simulink model "four_balloons"  (R2020b)
settings: Solver=VariableStepAuto  StartTime=0.0  StopTime=60*5  FixedStep=0.001  RelTol=1e-3
InitFcn:
  | seed1 = randi(100000);
  | seed2 = randi(200000);
model workspace (MAT data in the model file):
  dCoupling = 10
  kCoupling = 10
values from neighbouring files (symbols this model uses):
  Cd = a(4)    [comparisonPlot.m]    (also in optimiseB2.m = 0.185; optimiseBO.m = 0.185; params2.m = 0.185; sim_2balloon.m = 0.185)
  nH = x2nn.nH    [optimiseB2.m]    (also in optimiseBO.m = x.nH; params2.m = 10; sim_2balloon.m = x(2); sim_balloon.m = x(2))
  normalScaling = x2ll.normalScaling    [optimiseB2.m]    (also in optimiseBO.m = x.normalScaling; params2.m = 1; sim_2balloon.m = 0.259830816053; sim_balloon.m = x(5))
  nS = 1    [comparisonPlot.m]    (also in optimiseB2.m = x2nn.nS; optimiseBO.m = x.nS; params2.m = 0.025; sim_2balloon.m = x(3))
  nV = a(7)    [comparisonPlot.m]    (also in optimiseB2.m = x2nn.nV; optimiseBO.m = x.nV; params2.m = 0.5; sim_2balloon.m = x(1))
  rn = a(1)    [comparisonPlot.m]    (also in optimiseB2.m = 0.0625; optimiseBO.m = 0.0625; params2.m = 0.0625; sim_2balloon.m = 0.0625)
  seedX = randi(100000)    [optimiseB2.m]    (also in optimiseBO.m; params2.m; sim_2balloon.m; sim_balloon.m)
  seedX1 = randi(100000)    [optimiseB2.m]    (also in params2.m; sim_2balloon.m)
  seedY = randi(100000)    [optimiseB2.m]    (also in optimiseBO.m; params2.m; sim_2balloon.m; sim_balloon.m)
  seedY1 = randi(100000)    [optimiseB2.m]    (also in params2.m; sim_2balloon.m)
  seedZ = randi(100000)    [optimiseB2.m]    (also in optimiseBO.m; params2.m; sim_2balloon.m; sim_balloon.m)
  seedZ1 = randi(100000)    [optimiseB2.m]    (also in params2.m; sim_2balloon.m)
  theta = a(2)    [comparisonPlot.m]    (also in extract3D.m = deg2rad(-5); optimiseB2.m = x2ll.theta; optimiseBO.m = x.theta; params2.m = 3.5)
  V0 = a(3)    [comparisonPlot.m]    (also in optimiseB2.m = x2ll.V0; optimiseBO.m = x.V0; params2.m = 3.7; sim_2balloon.m = 1.01295922371)
libraries: nesl_utility x37, sm_lib x18, eeGeneralControl x12
(part 2 of 2)

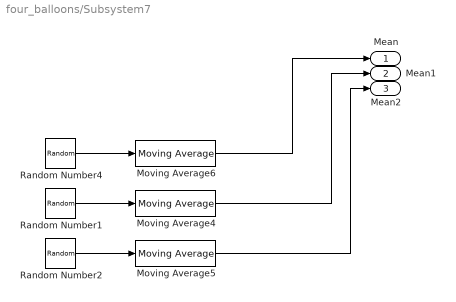
== system four_balloons/Subsystem7 ==
  Moving Average4 : eeGeneralControl/Moving Average  VariantControl=Variant1  LabelModeActiveChoice=Discrete  f=10  x0=0  Ts=nS/10
      settings: SourceProductBaseCode=PS
  Moving Average5 : eeGeneralControl/Moving Average  VariantControl=Variant1  LabelModeActiveChoice=Discrete  f=10  x0=0  Ts=nS/10
      settings: SourceProductBaseCode=PS
  Moving Average6 : eeGeneralControl/Moving Average  VariantControl=Variant1  LabelModeActiveChoice=Discrete  f=10  x0=0  Ts=nS/10
      settings: SourceProductBaseCode=PS
  Random Number1 : RandomNumber  Variance=nH  Seed=seedY1  SampleTime=nS
  Random Number2 : RandomNumber  Variance=nV  Seed=seedZ1  SampleTime=nS
  Random Number4 : RandomNumber  Variance=nH  Seed=seedX1  SampleTime=nS
  " Mean" : Outport
  " Mean1" : Outport  Port=2
  " Mean2" : Outport  Port=3
  wires:
  Moving Average4/1 -> " Mean1"/1
  Moving Average6/1 -> " Mean"/1
  Random Number4/1 -> Moving Average6/1
  Moving Average5/1 -> " Mean2"/1
  Random Number2/1 -> Moving Average5/1
  Random Number1/1 -> Moving Average4/1

== matlab function four_balloons/Subsystem6/Vertical dynamics ==
  data: fx output; sx output; fy output; sy output; x input; xdot input; y input; ydot input; z input; fz output; zdot input; parameters input; sz output

function [fx,sx,fy,sy,fz,sz] = fcn(x,xdot,y,ydot,z,zdot,parameters)

Cd = parameters(1);
rb = parameters(2);
rn = parameters(3);
theta = deg2rad(parameters(4)); 
V0 = parameters(5); 
normalScaling = parameters(6); 

%% Vertical forces

%Horizontal plane displacement
[rotation, rDisplacement] = cart2pol(x,y);

%flow radius
rFlow = rn+z*tan(theta);

%Peak flow velocity
meanFlowVelocity = V0*rn^2/(rFlow)^2;

%Velocity under ball
vFlowActual = flowSpeed(meanFlowVelocity,normalScaling*rFlow,rDisplacement);

%Relative
relativeVelocity = vFlowActual - zdot;

reZ = (1.22 * abs(relativeVelocity) * 2*rb)/(1.81*10^-5);

%Force
fz = sign(rFlow) * 0.5 * Cd * (pi * rb^2) * 1.22 * relativeVelocity^2;

%% Horizontal X forces

innerR = abs(x)-rb;
outerR = abs(x)+rb;
vInner = flowSpeed(meanFlowVelocity,normalScaling*rFlow,innerR);
vOuter = flowSpeed(meanFlowVelocity,normalScaling*rFlow,outerR);
fx = 0.5*1.22*(vOuter^2-vInner^2)*sign(x);

%% Horizontal Y forces
innerR = abs(y)-rb;%3*rb/8;
outerR = abs(y)+rb;%3*rb/8;
vInner = flowSpeed(meanFlowVelocity,normalScaling*rFlow,innerR);
vOuter = flowSpeed(meanFlowVelocity,normalScaling*rFlow,outerR);
fy = 0.5*1.22*(vOuter^2-vInner^2)*sign(y);

%% Drag
dragX = 0.5 * Cd * pi * rb^2 * 1.22 * xdot;
fx = fx - dragX;

dragY = 0.5 * Cd * pi * rb^2 * 1.22 * ydot;
fy = fy - dragY;

%% Force scalings
sx = flowSpeed(meanFlowVelocity,normalScaling*rFlow,x)/flowSpeed(meanFlowVelocity,rFlow,0);
sy = flowSpeed(meanFlowVelocity,normalScaling*rFlow,y)/flowSpeed(meanFlowVelocity,rFlow,0);
sz = flowSpeed(meanFlowVelocity,normalScaling*rFlow,rDisplacement)/flowSpeed(meanFlowVelocity,rFlow,0);

== matlab function four_balloons/Subsystem2/Vertical dynamics ==
  data: fx output; sx output; fy output; sy output; x input; xdot input; y input; ydot input; z input; fz output; zdot input; parameters input; sz output; relativeVelocity output
function [fx,sx,fy,sy,fz,sz, relativeVelocity] = fcn(x,xdot,y,ydot,z,zdot,parameters)

Cd = parameters(1);
rb = parameters(2);
rn = parameters(3);
theta = deg2rad(parameters(4)); 
V0 = parameters(5); 
normalScaling = parameters(6); 

%% Vertical forces

%Horizontal plane displacement
[rotation, rDisplacement] = cart2pol(x,y);

%flow radius
rFlow = rn+z*tan(theta);

%Peak flow velocity
meanFlowVelocity = V0*rn^2/(rFlow)^2;

%Velocity under ball
vFlowActual = flowSpeed(meanFlowVelocity,normalScaling*rFlow,rDisplacement);

%Relative
relativeVelocity = vFlowActual - zdot;

reZ = (1.22 * abs(relativeVelocity) * 2*rb)/(1.81*10^-5);

%Force
fz = sign(rFlow) * 0.5 * Cd * (pi * rb^2) * 1.22 * relativeVelocity^2;

%% Horizontal X forces

innerR = abs(x)-rb;
outerR = abs(x)+rb;
vInner = flowSpeed(meanFlowVelocity,normalScaling*rFlow,innerR);
vOuter = flowSpeed(meanFlowVelocity,normalScaling*rFlow,outerR);
fx = 0.5*1.22*(vOuter^2-vInner^2)*sign(x);

%% Horizontal Y forces
innerR = abs(y)-rb;%3*rb/8;
outerR = abs(y)+rb;%3*rb/8;
vInner = flowSpeed(meanFlowVelocity,normalScaling*rFlow,innerR);
vOuter = flowSpeed(meanFlowVelocity,normalScaling*rFlow,outerR);
fy = 0.5*1.22*(vOuter^2-vInner^2)*sign(y);

%% Drag
dragX = 0.5 * Cd * pi * rb^2 * 1.22 * xdot;
fx = fx - dragX;

dragY = 0.5 * Cd * pi * rb^2 * 1.22 * ydot;
fy = fy - dragY;

%% Force scalings
sx = flowSpeed(meanFlowVelocity,normalScaling*rFlow,x)/flowSpeed(meanFlowVelocity,rFlow,0);
sy = flowSpeed(meanFlowVelocity,normalScaling*rFlow,y)/flowSpeed(meanFlowVelocity,rFlow,0);
sz = flowSpeed(meanFlowVelocity,normalScaling*rFlow,rDisplacement)/flowSpeed(meanFlowVelocity,rFlow,0);

== matlab function four_balloons/Subsystem1/Vertical dynamics ==
  data: fx output; sx output; fy output; sy output; x input; xdot input; y input; ydot input; z input; fz output; zdot input; parameters input; sz output

function [fx,sx,fy,sy,fz,sz] = fcn(x,xdot,y,ydot,z,zdot,parameters)

Cd = parameters(1);
rb = parameters(2);
rn = parameters(3);
theta = deg2rad(parameters(4)); 
V0 = parameters(5); 
normalScaling = parameters(6); 

%% Vertical forces

%Horizontal plane displacement
[rotation, rDisplacement] = cart2pol(x,y);

%flow radius
rFlow = rn+z*tan(theta);

%Peak flow velocity
meanFlowVelocity = V0*rn^2/(rFlow)^2;

%Velocity under ball
vFlowActual = flowSpeed(meanFlowVelocity,normalScaling*rFlow,rDisplacement);

%Relative
relativeVelocity = vFlowActual - zdot;

reZ = (1.22 * abs(relativeVelocity) * 2*rb)/(1.81*10^-5);

%Force
fz = sign(rFlow) * 0.5 * Cd * (pi * rb^2) * 1.22 * relativeVelocity^2;

%% Horizontal X forces

innerR = abs(x)-rb;
outerR = abs(x)+rb;
vInner = flowSpeed(meanFlowVelocity,normalScaling*rFlow,innerR);
vOuter = flowSpeed(meanFlowVelocity,normalScaling*rFlow,outerR);
fx = 0.5*1.22*(vOuter^2-vInner^2)*sign(x);

%% Horizontal Y forces
innerR = abs(y)-rb;%3*rb/8;
outerR = abs(y)+rb;%3*rb/8;
vInner = flowSpeed(meanFlowVelocity,normalScaling*rFlow,innerR);
vOuter = flowSpeed(meanFlowVelocity,normalScaling*rFlow,outerR);
fy = 0.5*1.22*(vOuter^2-vInner^2)*sign(y);

%% Drag
dragX = 0.5 * Cd * pi * rb^2 * 1.22 * xdot;
fx = fx - dragX;

dragY = 0.5 * Cd * pi * rb^2 * 1.22 * ydot;
fy = fy - dragY;

%% Force scalings
sx = flowSpeed(meanFlowVelocity,normalScaling*rFlow,x)/flowSpeed(meanFlowVelocity,rFlow,0);
sy = flowSpeed(meanFlowVelocity,normalScaling*rFlow,y)/flowSpeed(meanFlowVelocity,rFlow,0);
sz = flowSpeed(meanFlowVelocity,normalScaling*rFlow,rDisplacement)/flowSpeed(meanFlowVelocity,rFlow,0);

== matlab function four_balloons/Subsystem4/Vertical dynamics ==
  data: fx output; sx output; fy output; sy output; x input; xdot input; y input; ydot input; z input; fz output; zdot input; parameters input; sz output

function [fx,sx,fy,sy,fz,sz] = fcn(x,xdot,y,ydot,z,zdot,parameters)

Cd = parameters(1);
rb = parameters(2);
rn = parameters(3);
theta = deg2rad(parameters(4)); 
V0 = parameters(5); 
normalScaling = parameters(6); 

%% Vertical forces

%Horizontal plane displacement
[rotation, rDisplacement] = cart2pol(x,y);

%flow radius
rFlow = rn+z*tan(theta);

%Peak flow velocity
meanFlowVelocity = V0*rn^2/(rFlow)^2;

%Velocity under ball
vFlowActual = flowSpeed(meanFlowVelocity,normalScaling*rFlow,rDisplacement);

%Relative
relativeVelocity = vFlowActual - zdot;

reZ = (1.22 * abs(relativeVelocity) * 2*rb)/(1.81*10^-5);

%Force
fz = sign(rFlow) * 0.5 * Cd * (pi * rb^2) * 1.22 * relativeVelocity^2;

%% Horizontal X forces

innerR = abs(x)-rb;
outerR = abs(x)+rb;
vInner = flowSpeed(meanFlowVelocity,normalScaling*rFlow,innerR);
vOuter = flowSpeed(meanFlowVelocity,normalScaling*rFlow,outerR);
fx = 0.5*1.22*(vOuter^2-vInner^2)*sign(x);

%% Horizontal Y forces
innerR = abs(y)-rb;%3*rb/8;
outerR = abs(y)+rb;%3*rb/8;
vInner = flowSpeed(meanFlowVelocity,normalScaling*rFlow,innerR);
vOuter = flowSpeed(meanFlowVelocity,normalScaling*rFlow,outerR);
fy = 0.5*1.22*(vOuter^2-vInner^2)*sign(y);

%% Drag
dragX = 0.5 * Cd * pi * rb^2 * 1.22 * xdot;
fx = fx - dragX;

dragY = 0.5 * Cd * pi * rb^2 * 1.22 * ydot;
fy = fy - dragY;

%% Force scalings
sx = flowSpeed(meanFlowVelocity,normalScaling*rFlow,x)/flowSpeed(meanFlowVelocity,rFlow,0);
sy = flowSpeed(meanFlowVelocity,normalScaling*rFlow,y)/flowSpeed(meanFlowVelocity,rFlow,0);
sz = flowSpeed(meanFlowVelocity,normalScaling*rFlow,rDisplacement)/flowSpeed(meanFlowVelocity,rFlow,0);
